simulink model "pendulo"  (R2020b)
settings: Solver=FixedStepDiscrete  StartTime=0.0  StopTime=Inf  FixedStep=0.001  RelTol=1e-3  EnableMultiTasking=on
libraries: arduinolib x2
settings Model: SimulationMode=external  SILPILModeSetting=veronly  ExtModeTrigDuration=2  Creator=aleca  LastModifiedBy=aleca
settings OptimizationCC: EnhancedBackFolding=on  PassReuseOutputArgsAs=Individual arguments  ZeroExternalMemoryAtStartup=off  ZeroInternalMemoryAtStartup=off  MaxStackSize=64  OptimizeBlockOrder=speed  DifferentSizesBufferReuse=on  OptimizationCustomize=off  EfficientTunableParamExpr=on
settings DebuggingCC: ParameterTunabilityLossMsg=error
settings HardwareCC: ProdBitPerInt=16  ProdBitPerPointer=16  ProdBitPerSizeT=16  ProdBitPerPtrDiffT=16  ProdLargestAtomicFloat=None  ProdWordSize=8  ProdHWDeviceType=Atmel->AVR  UseEmbeddedCoderFeatures=off  UseSimulinkCoderFeatures=off
settings SFSimCC: MATLABDynamicMemAlloc=off
settings RTWCC: Description=Embedded Coder  SystemTargetFile=ert.tlc  HardwareBoard=Arduino Mega 2560  TemplateMakefile=ert_default_tmf  RTWVerbose=off  Toolchain=Arduino AVR  BuildConfiguration=Faster Runs
settings CodeAppCC: ForceParamTrailComments=on  OperatorAnnotations=on  SimulinkDataObjDesc=on  SFDataObjDesc=on  MangleLength=10  InsertBlockDesc=on
settings ERTTargetCC: SupportContinuousTime=on  SupportNonInlinedSFcns=on  SupportVariableSizeSignals=on  ExtMode=on  ExtModeStaticAllocSize=2048  ExtModeMexArgs='127.0.0.1' 0 17725  ERTSrcFileBannerTemplate=codertarget_code_template.cgt  ERTHdrFileBannerTemplate=codertarget_code_template.cgt  ERTDataSrcFileTemplate=codertarget_code_template.cgt  ERTDataHdrFileTemplate=codertarget_code_template.cgt

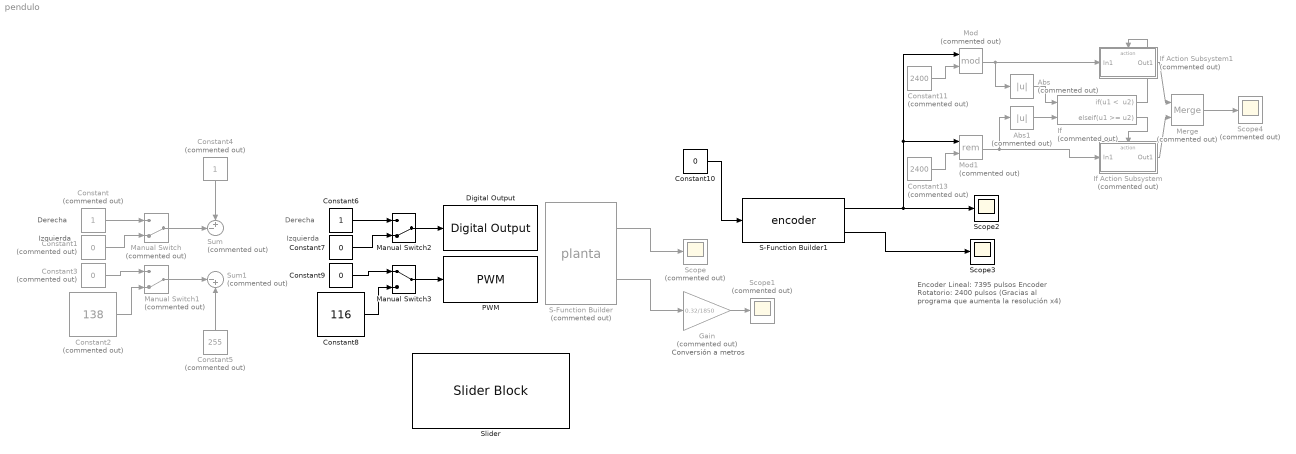
== system pendulo ==
  note: Encoder Lineal: 7395 pulsos
      | Encoder Rotatorio: 2400 pulsos
      | (Gracias al programa que aumenta la
      | resolución x4)
  note: Conversión a metros
  note: Derecha
  note: Izquierda
  note: Izquierda
  note: Derecha
  Abs : Abs  Commented=on
  Abs1 : Abs  Commented=on
  Constant : Constant  Commented=on  OutDataTypeStr=boolean  SampleTime=0.001
  Constant1 : Constant  Commented=on  Value=0  OutDataTypeStr=boolean  SampleTime=0.001
  Constant10 : Constant  Value=0  OutDataTypeStr=boolean  SampleTime=-1
  Constant11 : Constant  Commented=on  Value=2400  OutDataTypeStr=int16  SampleTime=-1
  Constant13 : Constant  Commented=on  Value=2400  OutDataTypeStr=int16  SampleTime=-1
  Constant2 : Constant  Commented=on  Value=138  OutDataTypeStr=int16  SampleTime=0.001
  Constant3 : Constant  Commented=on  Value=0  OutDataTypeStr=int16  SampleTime=0.001
  Constant4 : Constant  Commented=on  OutDataTypeStr=boolean  SampleTime=0.001
  Constant5 : Constant  Commented=on  Value=255  OutDataTypeStr=int16  SampleTime=-1
  Constant6 : Constant  OutDataTypeStr=boolean  SampleTime=0.001
  Constant7 : Constant  Value=0  OutDataTypeStr=boolean  SampleTime=0.001
  Constant8 : Constant  Value=116  OutDataTypeStr=int16  SampleTime=0.001
  Constant9 : Constant  Value=0  OutDataTypeStr=int16  SampleTime=0.001
  Digital Output : arduinolib/Digital Output  pinNumber=10  Direction=output  blockPlatform=arduino
  Gain : Gain  Commented=on  Gain=0.32/1850
  If : If  Commented=on  NumInputs=2  IfExpression="u1 <  u2"  ElseIfExpressions=u1 >= u2  ShowElse=off
  If Action Subsystem : Subsystem  Commented=on  TreatAsAtomicUnit=on
  If Action Subsystem1 : Subsystem  Commented=on  TreatAsAtomicUnit=on
  Manual Switch : ManualSwitch  Commented=on  CurrentSetting=0
  Manual Switch1 : ManualSwitch  Commented=on  CurrentSetting=0
  Manual Switch2 : ManualSwitch  CurrentSetting=0
  Manual Switch3 : ManualSwitch
  Merge : Merge  Commented=on
  Mod : Math  Commented=on  Operator=mod  SaturateOnIntegerOverflow=on
  Mod1 : Math  Commented=on  Operator=rem  SaturateOnIntegerOverflow=on
  PWM : arduinolib/PWM  pinNumber=9  frequencyType=Default  desiredFrequency=490.2  achievableFrequency=490.2
  S-Function Builder : S-Function  Commented=on  FunctionName=planta  SFunctionModules=planta_wrapper  SFunctionDeploymentMode=off  EnableBusSupport=off  mask(S-Function Builder){}
      mask help: Simulink:masks:SFunctionBuilder_MD
      mask init:
      | val = [[.9  0.75 0.75 1 1 .9 .9 1]',[1 1 0.75 0.75 .9 .9 1 .9]'];try , sys = get_param(gcb,'SfunBuilderFcnName');if isempty(sys), sys = get_param(gcb,'FunctionName'); end,catch, sys = get_param(gcb,'FunctionName'); end
      settings: CopyFcn=set_param(gcbh,'LinkStatus','none')  OpenFcn=sfunctionwizard(gcbh)
      mask Display:
      | plot(val(:,1),val(:,2))
      | disp(sys)
      | port_label('output',1,'rotPos_OUT')
      | port_label('output',2,'linPosOut_OUT')
  S-Function Builder1 : S-Function  FunctionName=encoder  SFunctionModules=encoder_wrapper  SFunctionDeploymentMode=off  EnableBusSupport=off  mask(S-Function Builder){}
      mask help: Simulink:masks:SFunctionBuilder_MD
      mask init: same as pendulo/S-Function Builder
      settings: CopyFcn=set_param(gcbh,'LinkStatus','none')  OpenFcn=sfunctionwizard(gcbh)
      mask Display:
      | plot(val(:,1),val(:,2))
      | disp(sys)
      | port_label('input',1,'reset')
      | port_label('output',1,'rotpos')
      | port_label('output',2,'linpos')
  Scope : Scope  Commented=on
  Scope1 : Scope  Commented=on
  Scope2 : Scope
  Scope3 : Scope
  Scope4 : Scope  Commented=on
  Slider : SliderBlock  ScaleMax=255  TickInterval=2
  Sum : Sum  Commented=on  Inputs=+-|
  Sum1 : Sum  Commented=on  Inputs=|-+
  wires:
  Constant/1 -> Manual Switch/1
  Constant1/1 -> Manual Switch/2
  Constant3/1 -> Manual Switch1/1
  Constant2/1 -> Manual Switch1/2
  Gain/1 -> Scope1/1
  Constant4/1 -> Sum/1
  Manual Switch/1 -> Sum/2
  Manual Switch1/1 -> Sum1/1
  Constant5/1 -> Sum1/2
  Constant7/1 -> Manual Switch2/2
  Constant6/1 -> Manual Switch2/1
  Constant8/1 -> Manual Switch3/2
  Constant9/1 -> Manual Switch3/1
  Manual Switch2/1 -> Digital Output/1
  Manual Switch3/1 -> PWM/1
  S-Function Builder/1 -> Scope/1
  S-Function Builder/2 -> Gain/1
  S-Function Builder1/2 -> Scope3/1
  Constant10/1 -> S-Function Builder1/1
  Mod1/1 -> If Action Subsystem/1(In1), Abs1/1
  If/1 -> If Action Subsystem1/Action
  If/2 -> If Action Subsystem/Action
  If Action Subsystem/1(Out1) -> Merge/2
  If Action Subsystem1/1(Out1) -> Merge/1
  Mod/1 -> If Action Subsystem1/1(In1), Abs/1
  Constant11/1 -> Mod/2
  S-Function Builder1/1 -> Scope2/1, Mod1/1, Mod/1
  Constant13/1 -> Mod1/2
  Merge/1 -> Scope4/1
  Abs/1 -> If/1
  Abs1/1 -> If/2

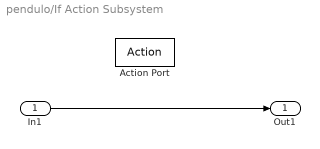
== system pendulo/If Action Subsystem ==
  In1 : Inport
  Action Port : ActionPort  ActionPortLabel=elseif(u1 >= u2)
  Out1 : Outport
  wires:
  In1/1 -> Out1/1

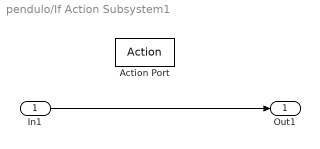
== system pendulo/If Action Subsystem1 ==
  In1 : Inport
  Action Port : ActionPort  ActionPortLabel="if(u1 <  u2)"
  Out1 : Outport
  wires:
  In1/1 -> Out1/1
